simulink model "manualstartTraj"  (R2016a)
settings: Solver=ode5  StartTime=0.0  StopTime=inf  FixedStep=0.001  RelTol=1e-3
undefined symbols (not defined in the file): dt, qraw_trans
libraries: simulink x4
settings Model: SimulationMode=external  Creator=julianleland  LastModifiedBy=julianleland
settings HardwareCC: ProdBitPerLong=64  ProdLargestAtomicFloat=None  ProdHWDeviceType=Intel->x86-64  TargetBitPerLong=64  TargetBitPerPointer=64  TargetIntDivRoundTo=Zero  TargetEndianess=LittleEndian  TargetWordSize=64  TargetHWDeviceType=Intel->x86-64
settings RTWCC: SystemTargetFile=sldrt.tlc  TemplateMakefile=sldrt.tmf  Description=Simulink Desktop Real-Time  RTWCompilerOptimization=on
settings CodeAppCC: MaxIdLength=95
settings SimulinkDesktopRealTimeCC: TargetPreCompLibLocation=/Applications/MATLAB_R2016a.app/toolbox/sldrt/lib/maci64  TargetLangStandard=C89/C90 (ANSI)  SupportVariableSizeSignals=off

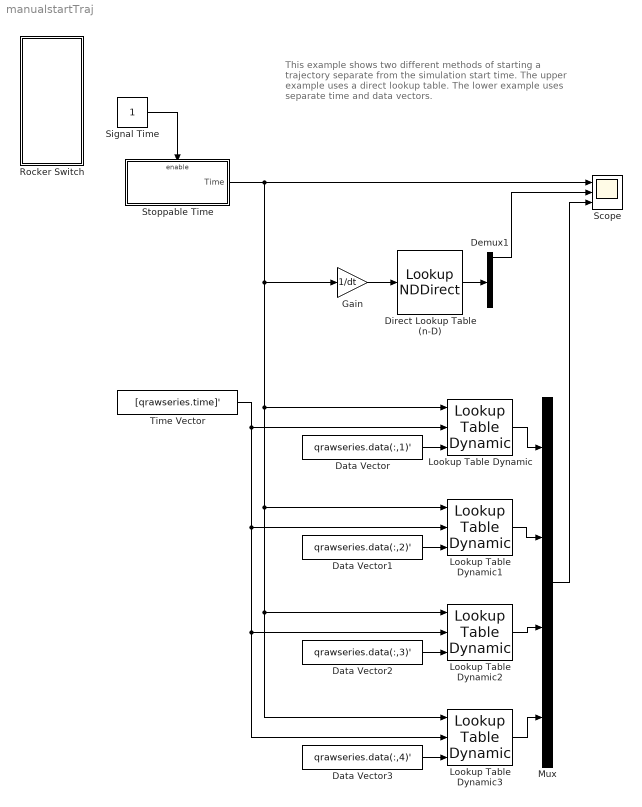
== system manualstartTraj ==
  note: This example shows two different methods of starting a trajectory separate from the simulation start time. The upper example uses a direct lookup table. The lower example uses separate time and data vectors.
  Data Vector : FromWorkspace  VariableName=qrawseries.data(:,1)'  SampleTime=0
  Data Vector1 : FromWorkspace  VariableName=qrawseries.data(:,2)'  SampleTime=0
  Data Vector2 : FromWorkspace  VariableName=qrawseries.data(:,3)'  SampleTime=0
  Data Vector3 : FromWorkspace  VariableName=qrawseries.data(:,4)'  SampleTime=0
  Demux1 : Demux
  Direct Lookup Table (n-D) : LookupNDDirect  InputsSelectThisObjectFromTable=Column  Table=qraw_trans
  Gain : Gain  Gain=1/dt
  Lookup Table Dynamic{,1..3} (4 alike) : simulink/Lookup Tables/Lookup Table Dynamic  LookUpMeth=Interpolation-Use End Values  OutDataTypeStr=Inherit: Inherit via back propagation  OutDataType=fixdt('double')  OutScaling=2^-10  DoSatur=off
  Mux : Mux
  Rocker Switch : Subsystem  DialogController=hmiCreateDDGDialog  IsWebBlock=on  mask(MWDashboardBlock){webBlockId=1de22ea1-65b7-4644-8b2d-3f138c4c2673, webBlockType=rockerswitch, ShowInLibBrowser=on, ShowInitialText=on, HMISrcModelName=manualstartTraj}
      mask prompts: webBlockId "WebBlock Id"; webBlockType "WebBlock Type"; HMISrcModelName "Source Model"
      mask Help: helpview([docroot '/mapfiles/simulink.map'], 'hmi_rocker_switch')
      mask Display:
      | if strcmp(get_param(bdroot(gcb),'BlockDiagramType'), 'library')
      |     image([(matlabroot) '/toolbox/simulink/hmi/icons/RockerSwitch.png']);
      | end
  Scope : Scope  NumInputPorts=3
  Signal Time : Constant
  Stoppable Time : Subsystem  TreatAsAtomicUnit=on
  Time Vector : FromWorkspace  VariableName=[qrawseries.time]'  SampleTime=0
  wires:
  Signal Time/1 -> Stoppable Time/Enable
  Stoppable Time/1(Time) -> Gain/1, Lookup Table Dynamic3/1, Lookup Table Dynamic2/1, Lookup Table Dynamic1/1, Lookup Table Dynamic/1, Scope/1
  Gain/1 -> Direct Lookup Table (n-D)/1
  Time Vector/1 -> Lookup Table Dynamic1/2, Lookup Table Dynamic3/2, Lookup Table Dynamic2/2, Lookup Table Dynamic/2
  Direct Lookup Table (n-D)/1 -> Demux1/1
  Demux1/1 -> Scope/2
  Data Vector/1 -> Lookup Table Dynamic/3
  Data Vector1/1 -> Lookup Table Dynamic1/3
  Data Vector2/1 -> Lookup Table Dynamic2/3
  Data Vector3/1 -> Lookup Table Dynamic3/3
  Lookup Table Dynamic3/1 -> Mux/4
  Lookup Table Dynamic2/1 -> Mux/3
  Lookup Table Dynamic1/1 -> Mux/2
  Lookup Table Dynamic/1 -> Mux/1
  Mux/1 -> Scope/3

== system manualstartTraj/Rocker Switch ==

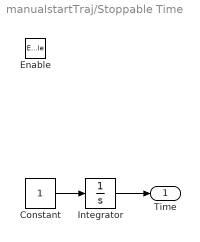
== system manualstartTraj/Stoppable Time ==
  Enable : EnablePort
  Constant : Constant
  Integrator : Integrator
  Time : Outport
  wires:
  Constant/1 -> Integrator/1
  Integrator/1 -> Time/1
